simulink model "t2h_TestBed1_org"  (Simulink 10.0)
settings: Solver=FixedStepDiscrete  StartTime=0.0  StopTime=1  FixedStep=1  RelTol=1e-3  EnableMultiTasking=on
undefined symbols (not defined in the file): MWS
libraries: Lib_Thermo_Temp2Enth_TMATS x1
settings Model: Creator=jwchapm2  LastModifiedBy=bhisma
settings DataIOCC: LimitDataPoints=on
settings OptimizationCC: ExpressionDepthLimit=2147483647
settings DebuggingCC: SolverPrmCheckMsg=warning  StateNameClashWarn=warning
settings GRTTargetCC: GeneratePreprocessorConditionals=Disable all  CombineOutputUpdateFcns=on  GRTInterface=off
settings ConfigComp: CovExternalEMLEnable=off

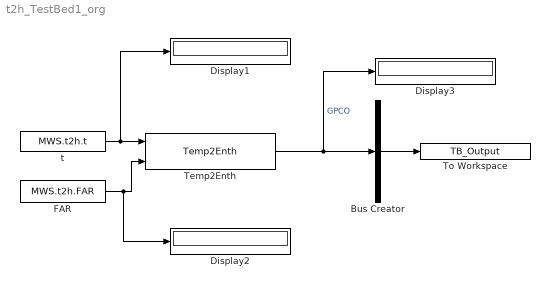
== system t2h_TestBed1_org ==
  Bus Creator : BusCreator  Inputs=1
  Display1 : Display
  Display2 : Display
  Display3 : Display
  FAR : Constant  Value=MWS.t2h.FAR
  Temp2Enth : Lib_Thermo_Temp2Enth_TMATS/Temp2Enth
  To Workspace : ToWorkspace  VariableName=TB_Output  SampleTime=-1
  t : Constant  Value=MWS.t2h.t
  wires:
  FAR/1 -> Display2/1, Temp2Enth/2
  t/1 -> Display1/1, Temp2Enth/1
  Temp2Enth/1 -> Display3/1, Bus Creator/1  "GPCO"
  Bus Creator/1 -> To Workspace/1
